simulink model "bh_zaz"  (R2016b)
settings: Solver=ode23s  StartTime=0.0  StopTime=15  RelTol=1e-5  EnableMultiTasking=on
undefined symbols (not defined in the file or in its folder): b1_damp, b2_damp, g, I1g, I2g, L1x, L1y, L1z, L2x, L2y, L2z, mass1, mass2, theta1_0, theta1_dot_0, theta2_0, theta2_dot_0, X, Y, Z
libraries: sm_lib x11, nesl_utility x10
settings Model: Creator=bhorton  LastModifiedBy=bhorton
settings SolverCC: ZeroCrossAlgorithm=Adaptive
settings OptimizationCC: LifeSpan=inf
settings DebuggingCC: SFUnexpectedBacktrackingDiag=warning  SFNoUnconditionalDefaultTransitionDiag=warning  SFExecutionAtInitializationDiag=none
settings GRTTargetCC: TargetLangStandard=C89/C90 (ANSI)
settings ConfigComp: CovMetricSettings=dw  CovHtmlReporting=on  CovSaveCumulativeToWorkspaceVar=on  CovSaveSingleToWorkspaceVar=on  CovExternalEMLEnable=off
settings SimscapeCC: SimscapeLogType=all  SimscapeLogDataHistory=10000

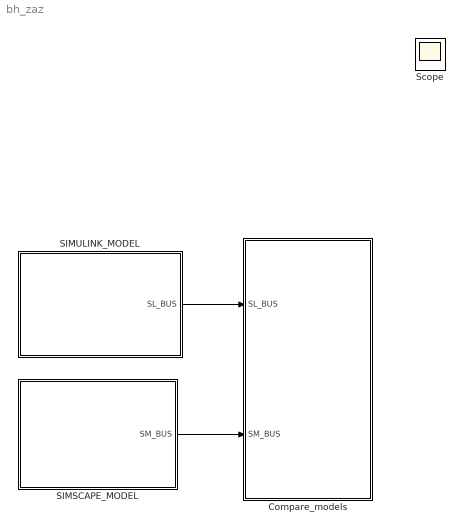
== system bh_zaz ==
  Compare_models : Subsystem
  SIMSCAPE_MODEL : Subsystem
  SIMULINK_MODEL : Subsystem
  Scope : Scope
  wires:
  SIMULINK_MODEL/1(SL_BUS) -> Compare_models/1(SL_BUS)
  SIMSCAPE_MODEL/1(SM_BUS) -> Compare_models/2(SM_BUS)

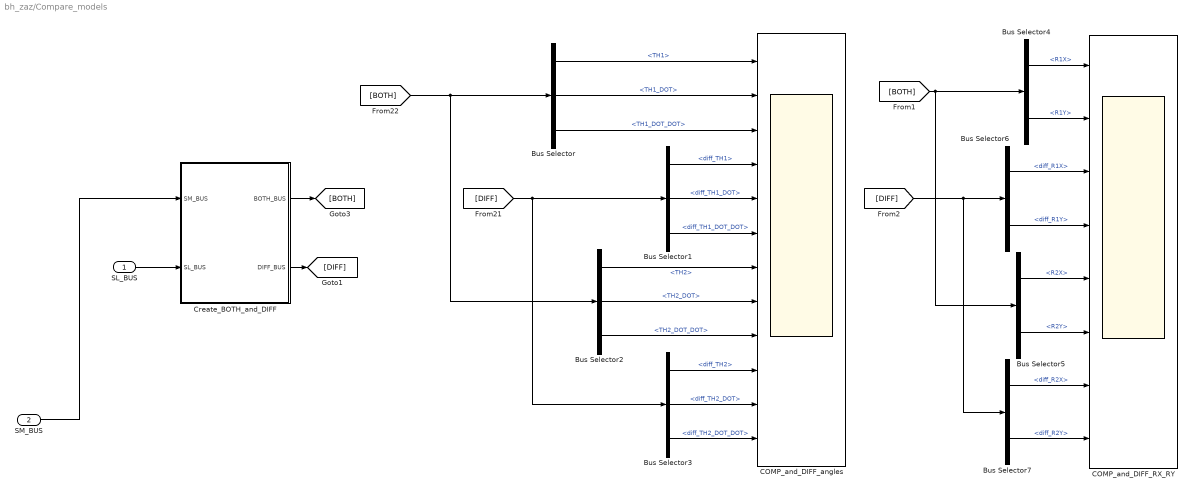
== system bh_zaz/Compare_models ==
  SL_BUS : Inport
  SM_BUS : Inport  Port=2
  Bus Selector : BusSelector  OutputSignals=TH1,TH1_DOT,TH1_DOT_DOT
  Bus Selector1 : BusSelector  OutputSignals=diff_TH1,diff_TH1_DOT,diff_TH1_DOT_DOT
  Bus Selector2 : BusSelector  OutputSignals=TH2,TH2_DOT,TH2_DOT_DOT
  Bus Selector3 : BusSelector  OutputSignals=diff_TH2,diff_TH2_DOT,diff_TH2_DOT_DOT
  Bus Selector4 : BusSelector  OutputSignals=R1X,R1Y
  Bus Selector5 : BusSelector  OutputSignals=R2X,R2Y
  Bus Selector6 : BusSelector  OutputSignals=diff_R1X,diff_R1Y
  Bus Selector7 : BusSelector  OutputSignals=diff_R2X,diff_R2Y
  COMP_and_DIFF_RX_RY : Scope  NumInputPorts=8
  COMP_and_DIFF_angles : Scope  NumInputPorts=12
  Create_BOTH_and_DIFF : Subsystem
  wires:
  SM_BUS/1 -> Create_BOTH_and_DIFF/1(SM_BUS)
  Bus Selector/3 -> COMP_and_DIFF_angles/3  "<TH1_DOT_DOT>"
  Bus Selector/2 -> COMP_and_DIFF_angles/2  "<TH1_DOT>"
  Bus Selector/1 -> COMP_and_DIFF_angles/1  "<TH1>"
  SL_BUS/1 -> Create_BOTH_and_DIFF/2(SL_BUS)
  Bus Selector1/1 -> COMP_and_DIFF_angles/4  "<diff_TH1>"
  Bus Selector1/2 -> COMP_and_DIFF_angles/5  "<diff_TH1_DOT>"
  Bus Selector1/3 -> COMP_and_DIFF_angles/6  "<diff_TH1_DOT_DOT>"
  Bus Selector2/1 -> COMP_and_DIFF_angles/7  "<TH2>"
  Bus Selector2/2 -> COMP_and_DIFF_angles/8  "<TH2_DOT>"
  Bus Selector2/3 -> COMP_and_DIFF_angles/9  "<TH2_DOT_DOT>"
  Bus Selector3/1 -> COMP_and_DIFF_angles/10  "<diff_TH2>"
  Bus Selector3/2 -> COMP_and_DIFF_angles/11  "<diff_TH2_DOT>"
  Bus Selector3/3 -> COMP_and_DIFF_angles/12  "<diff_TH2_DOT_DOT>"
  Create_BOTH_and_DIFF/1(BOTH_BUS) -> [BOTH]
  Create_BOTH_and_DIFF/2(DIFF_BUS) -> [DIFF]
  [BOTH] -> Bus Selector2/1, Bus Selector/1
  [DIFF] -> Bus Selector1/1, Bus Selector3/1
  Bus Selector4/2 -> COMP_and_DIFF_RX_RY/2  "<R1Y>"
  Bus Selector4/1 -> COMP_and_DIFF_RX_RY/1  "<R1X>"
  [BOTH] -> Bus Selector4/1, Bus Selector5/1
  Bus Selector5/1 -> COMP_and_DIFF_RX_RY/5  "<R2X>"
  Bus Selector5/2 -> COMP_and_DIFF_RX_RY/6  "<R2Y>"
  [DIFF] -> Bus Selector7/1, Bus Selector6/1
  Bus Selector6/1 -> COMP_and_DIFF_RX_RY/3  "<diff_R1X>"
  Bus Selector6/2 -> COMP_and_DIFF_RX_RY/4  "<diff_R1Y>"
  Bus Selector7/1 -> COMP_and_DIFF_RX_RY/7  "<diff_R2X>"
  Bus Selector7/2 -> COMP_and_DIFF_RX_RY/8  "<diff_R2Y>"

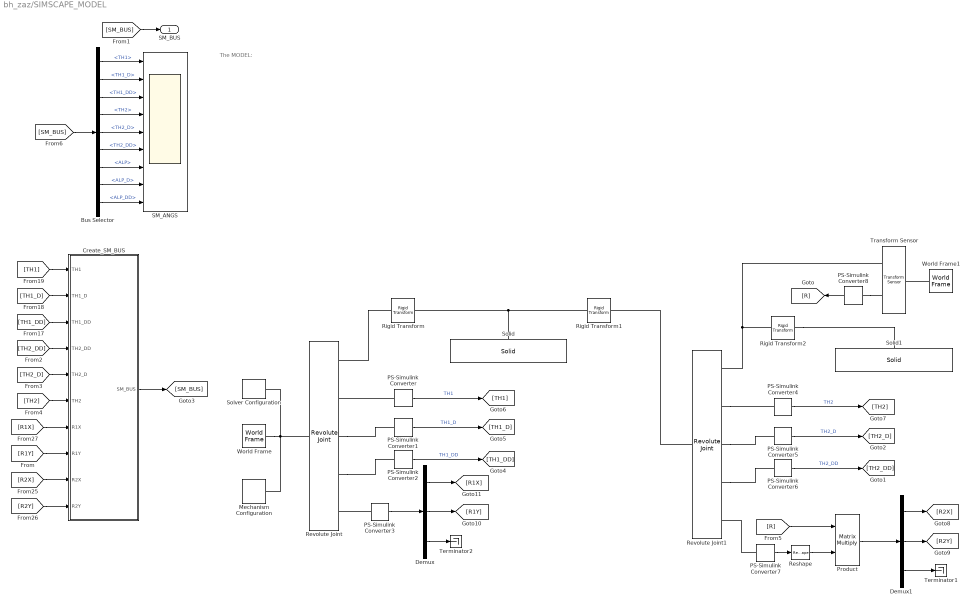
== system bh_zaz/SIMSCAPE_MODEL ==
  note: The MODEL:
  Bus Selector : BusSelector  OutputSignals=TH1,TH1_D,TH1_DD,TH2,TH2_D,TH2_DD,ALP,ALP_D,ALP_DD
  Create_SM_BUS : Subsystem
  Demux : Demux  Outputs=3
  Demux1 : Demux  Outputs=3
  Mechanism Configuration : sm_lib/Utilities/Mechanism Configuration  UniformGravity=Constant  GravityVector=[0 -9.80665 0 ]  GravityUnits=m/s^2  LinearizationDelta=0.001
  PS-Simulink Converter : nesl_utility/PS-Simulink Converter  PhysicalDomain=network_engine_domain  SubClassName=ps_output  LeftPortType=input  RightPortType=output  PseudoPeriodic=off  Frequencies=[]  Unit=rad  AffineConversion=off
  PS-Simulink Converter1 : nesl_utility/PS-Simulink Converter  PhysicalDomain=network_engine_domain  SubClassName=ps_output  LeftPortType=input  RightPortType=output  PseudoPeriodic=off  Frequencies=[]  Unit=rad/s  AffineConversion=off
  PS-Simulink Converter2 : nesl_utility/PS-Simulink Converter  PhysicalDomain=network_engine_domain  SubClassName=ps_output  LeftPortType=input  RightPortType=output  PseudoPeriodic=off  Frequencies=[]  Unit=rad/s^2  AffineConversion=off
  PS-Simulink Converter3 : nesl_utility/PS-Simulink Converter  PhysicalDomain=network_engine_domain  SubClassName=ps_output  LeftPortType=input  RightPortType=output  PseudoPeriodic=off  Frequencies=[]  Unit=N  AffineConversion=off
  PS-Simulink Converter4 : nesl_utility/PS-Simulink Converter  PhysicalDomain=network_engine_domain  SubClassName=ps_output  LeftPortType=input  RightPortType=output  PseudoPeriodic=off  Frequencies=[]  Unit=rad  AffineConversion=off
  PS-Simulink Converter5 : nesl_utility/PS-Simulink Converter  PhysicalDomain=network_engine_domain  SubClassName=ps_output  LeftPortType=input  RightPortType=output  PseudoPeriodic=off  Frequencies=[]  Unit=rad/s  AffineConversion=off
  PS-Simulink Converter6 : nesl_utility/PS-Simulink Converter  PhysicalDomain=network_engine_domain  SubClassName=ps_output  LeftPortType=input  RightPortType=output  PseudoPeriodic=off  Frequencies=[]  Unit=rad/s^2  AffineConversion=off
  PS-Simulink Converter7 : nesl_utility/PS-Simulink Converter  PhysicalDomain=network_engine_domain  SubClassName=ps_output  LeftPortType=input  RightPortType=output  PseudoPeriodic=off  Frequencies=[]  Unit=N  AffineConversion=off
  PS-Simulink Converter8 : nesl_utility/PS-Simulink Converter  PhysicalDomain=network_engine_domain  SubClassName=ps_output  LeftPortType=input  RightPortType=output  PseudoPeriodic=off  Frequencies=[]  Unit=1  AffineConversion=off
  Product : Product  Multiplication=Matrix(*)
  Reshape : Reshape  OutputDimensionality=Column vector (2-D)
  Revolute Joint : sm_lib/Joints/Revolute Joint  SenseConstraintForce=on  SenseConstraintForceX=off  SenseConstraintForceY=off  SenseConstraintForceZ=off  SenseConstraintTorque=off  SenseConstraintTorqueX=off  SenseConstraintTorqueY=off  SenseConstraintTorqueZ=off  SenseTotalForce=off  SenseTotalForceX=off  SenseTotalForceY=off  SenseTotalForceZ=off  SenseTotalTorque=off  SenseTotalTorqueX=off  SenseTotalTorqueY=off  SenseTotalTorqueZ=off  CompositeWrenchDir=BaseOnFollower  CompositeWrenchFrame=BaseFrame  EquilibriumPosition=0  EquilibriumPositionUnits=deg  SpringStiffness=0  SpringStiffnessUnits=N*m/deg  DampingCoefficient=b1_damp  DampingCoefficientUnits=N*m/(rad/s)  TorqueActuationMode=NoTorque  MotionActuationMode=ComputedMotion  SensePosition=on  SenseVelocity=on  SenseAcceleration=on  SenseTorqueForce=off  PositionTargetSpecify=on  PositionTargetPriority=Low  PositionTargetValue=theta1_0  PositionTargetValueUnits=rad  VelocityTargetSpecify=on  VelocityTargetPriority=High  VelocityTargetValue=theta1_dot_0  VelocityTargetValueUnits=rad/s
  Revolute Joint1 : sm_lib/Joints/Revolute Joint  SenseConstraintForce=on  SenseConstraintForceX=off  SenseConstraintForceY=off  SenseConstraintForceZ=off  SenseConstraintTorque=off  SenseConstraintTorqueX=off  SenseConstraintTorqueY=off  SenseConstraintTorqueZ=off  SenseTotalForce=off  SenseTotalForceX=off  SenseTotalForceY=off  SenseTotalForceZ=off  SenseTotalTorque=off  SenseTotalTorqueX=off  SenseTotalTorqueY=off  SenseTotalTorqueZ=off  CompositeWrenchDir=BaseOnFollower  CompositeWrenchFrame=FollowerFrame  EquilibriumPosition=0  EquilibriumPositionUnits=deg  SpringStiffness=0  SpringStiffnessUnits=N*m/deg  DampingCoefficient=b2_damp  DampingCoefficientUnits=N*m/(rad/s)  TorqueActuationMode=NoTorque  MotionActuationMode=ComputedMotion  SensePosition=on  SenseVelocity=on  SenseAcceleration=on  SenseTorqueForce=off  PositionTargetSpecify=on  PositionTargetPriority=Low  PositionTargetValue=theta2_0  PositionTargetValueUnits=rad  VelocityTargetSpecify=on  VelocityTargetPriority=High  VelocityTargetValue=theta2_dot_0  VelocityTargetValueUnits=rad/s
  Rigid Transform : sm_lib/Frames and Transforms/Rigid Transform  TranslationMethod=StandardAxis  TranslationStandardOffset=L1x/2  TranslationLengthUnit=m  TranslationStandardAxis=+X  TranslationCartesianOffset=[0 0 0]  TranslationROffset=0  TranslationROffsetUnits=m  TranslationZOffset=0  TranslationZOffsetUnits=m  TranslationThetaOffset=0  TranslationThetaOffsetUnits=deg  RotationMethod=None  RotationAngleUnits=deg  RotationStandardAxis=+Z  RotationAngle=0.0  RotationArbitraryAxis=[0 0 1]  FollAlignAxisA=+X  BaseAlignAxisA=+Y  FollAlignAxisB=+Y  BaseAlignAxisB=+Z  RotationSequenceAxes=FollowerAxes  RotationSequence=XYX  RotationSequenceAngles=[0 0 0]  RotationSequenceAnglesUnits=deg  RotationMatrix=[1 0 0; 0 1 0; 0 0 1]
  Rigid Transform1 : sm_lib/Frames and Transforms/Rigid Transform  TranslationMethod=StandardAxis  TranslationStandardOffset=L1x/2  TranslationLengthUnit=m  TranslationStandardAxis=+X  TranslationCartesianOffset=[0 0 0]  TranslationROffset=0  TranslationROffsetUnits=m  TranslationZOffset=0  TranslationZOffsetUnits=m  TranslationThetaOffset=0  TranslationThetaOffsetUnits=deg  RotationMethod=None  RotationAngleUnits=deg  RotationStandardAxis=+Z  RotationAngle=0.0  RotationArbitraryAxis=[0 0 1]  FollAlignAxisA=+X  BaseAlignAxisA=+Y  FollAlignAxisB=+Y  BaseAlignAxisB=+Z  RotationSequenceAxes=FollowerAxes  RotationSequence=XYX  RotationSequenceAngles=[0 0 0]  RotationSequenceAnglesUnits=deg  RotationMatrix=[1 0 0; 0 1 0; 0 0 1]
  Rigid Transform2 : sm_lib/Frames and Transforms/Rigid Transform  TranslationMethod=StandardAxis  TranslationStandardOffset=L2x/2  TranslationLengthUnit=m  TranslationStandardAxis=+X  TranslationCartesianOffset=[0 0 0]  TranslationROffset=0  TranslationROffsetUnits=m  TranslationZOffset=0  TranslationZOffsetUnits=m  TranslationThetaOffset=0  TranslationThetaOffsetUnits=deg  RotationMethod=None  RotationAngleUnits=deg  RotationStandardAxis=+Z  RotationAngle=0.0  RotationArbitraryAxis=[0 0 1]  FollAlignAxisA=+X  BaseAlignAxisA=+Y  FollAlignAxisB=+Y  BaseAlignAxisB=+Z  RotationSequenceAxes=FollowerAxes  RotationSequence=XYX  RotationSequenceAngles=[0 0 0]  RotationSequenceAnglesUnits=deg  RotationMatrix=[1 0 0; 0 1 0; 0 0 1]
  SM_ANGS : Scope  NumInputPorts=9
  Solid : sm_lib/Body Elements/Solid  InertiaType=CalculateFromGeometry  Mass=1  MassUnits=kg  CenterOfMass=[0 0 0]  CenterOfMassUnits=m  MomentsOfInertia=[1 1 1]  MomentsOfInertiaUnits=kg*m^2  ProductsOfInertia=[0 0 0]  ProductsOfInertiaUnits=kg*m^2  DensityBased=on  Density=density  DensityUnits=kg/(m^3)  DoExposeReferenceFrame=on  SerializedFrames=<Frames/>  GraphicType=FromGeometry  MarkerShape=Sphere  MarkerSize=10  GraphicVisPropType=SimpleVisualProperties  GraphicDiffuseColor=[0.8 0.8 1.0]  GraphicSpecularColor=[0.5 0.5 0.5 1.0]  GraphicAmbientColor=[0.15 0.15 0.15 1.0]  GraphicEmissiveColor=[0.0 0.0 0.0 1.0]  GraphicShininess=75  GraphicOpacity=1.0  GeometryShape=Brick  RectangleSize=[1 1]  RectangleSizeUnits=m  BrickDimensions=[L1x, L1y, L1z ]  BrickDimensionUnits=m  CylinderRadius=1  CylinderRadiusUnits=m  CylinderLength=1  CylinderLengthUnits=m  SphereRadius=1  SphereRadiusUnits=m  EllipsoidRadii=[1 1 1]  EllipsoidRadiiUnits=m  ExtrusionCrossSection=[1 1; -1 1; -1 -1; 1 -1]  ExtrusionCrossSectionUnits=m  ExtrusionLength=1  ExtrusionLengthUnits=m  PolygonNumSides=3  PolygonOuterRadius=1  PolygonOuterRadiusUnits=m  ExtGeomFileType=STEP  ExtGeomFileUnits=m  RevolutionCrossSection=[1 1; 1 -1; 2 -1; 2 1]  RevolutionCrossSectionUnits=m  RevolutionExtent=Full  RevolutionAngle=180  RevolutionAngleUnits=deg
  Solid1 : sm_lib/Body Elements/Solid  InertiaType=CalculateFromGeometry  Mass=1  MassUnits=kg  CenterOfMass=[0 0 0]  CenterOfMassUnits=m  MomentsOfInertia=[1 1 1]  MomentsOfInertiaUnits=kg*m^2  ProductsOfInertia=[0 0 0]  ProductsOfInertiaUnits=kg*m^2  DensityBased=on  Density=density  DensityUnits=kg/(m^3)  DoExposeReferenceFrame=on  SerializedFrames=<Frames/>  GraphicType=FromGeometry  MarkerShape=Sphere  MarkerSize=10  GraphicVisPropType=SimpleVisualProperties  GraphicDiffuseColor=[1.0 0.6 1.0]  GraphicSpecularColor=[0.5 0.5 0.5 1.0]  GraphicAmbientColor=[0.15 0.15 0.15 1.0]  GraphicEmissiveColor=[0.0 0.0 0.0 1.0]  GraphicShininess=75  GraphicOpacity=1.0  GeometryShape=Brick  RectangleSize=[1 1]  RectangleSizeUnits=m  BrickDimensions=[L2x, L2y, L2z ]  BrickDimensionUnits=m  CylinderRadius=1  CylinderRadiusUnits=m  CylinderLength=1  CylinderLengthUnits=m  SphereRadius=1  SphereRadiusUnits=m  EllipsoidRadii=[1 1 1]  EllipsoidRadiiUnits=m  ExtrusionCrossSection=[1 1; -1 1; -1 -1; 1 -1]  ExtrusionCrossSectionUnits=m  ExtrusionLength=1  ExtrusionLengthUnits=m  PolygonNumSides=3  PolygonOuterRadius=1  PolygonOuterRadiusUnits=m  ExtGeomFileType=STEP  ExtGeomFileUnits=m  RevolutionCrossSection=[1 1; 1 -1; 2 -1; 2 1]  RevolutionCrossSectionUnits=m  RevolutionExtent=Full  RevolutionAngle=180  RevolutionAngleUnits=deg
  Solver Configuration : nesl_utility/Solver Configuration  PhysicalDomain=network_engine_domain  SubClassName=solver  LeftPortType=input  RightPortType=generic  Accelerate=off  Tones=[]  Harmonics=[]  SimulateNoise=off  Profile=off  UseLocalSampling=off  EnableSwitchedLinearOptims=on  FrequencyDomain=off  UseCCode=off  RelTol=0.001  AbsTol=1e-06  MinStep=1e-09  ToWorkspace=off  RevertToSquareIcSolve=off  NumHomotopyIterations=100  PhasorMode=off  PhasorModeNumHarmonics=1  OverrideAbsTol=off  DoDC=off  ResidualTolerance=1e-09  UseLocalSolver=off  LocalSolverChoice=NE_BACKWARD_EULER_ADVANCER  LocalSolverSampleTime=0.001  DoFixedCost=off  MaxNonlinIter=3  MaxModeIter=2  LinearAlgebra=Sparse  DelaysMemoryBudget=1024  AutomaticFiltering=on  FilteringTimeConstant=0.001
  Terminator1 : Terminator
  Terminator2 : Terminator
  Transform Sensor : sm_lib/Frames and Transforms/Transform Sensor  MeasurementFrame=World  SenseAngle=off  SenseAxis=off  SenseAngle1=off  SenseAngle2=off  SenseAngle3=off  SenseQ=off  SenseR=on  SenseOmegaX=off  SenseOmegaY=off  SenseOmegaZ=off  SenseOmega1=off  SenseOmega2=off  SenseOmega3=off  SenseQDot=off  SenseRDot=off  SenseAlphaX=off  SenseAlphaY=off  SenseAlphaZ=off  SenseAlpha1=off  SenseAlpha2=off  SenseAlpha3=off  SenseQDDot=off  SenseRDDot=off  SenseX=off  SenseY=off  SenseZ=off  SenseRad=off  SenseAzim=off  SenseDist=off  SenseInc=off  SenseXDot=off  SenseYDot=off  SenseZDot=off  SenseRadDot=off  SenseAzimDot=off  SenseDistDot=off  SenseIncDot=off  SenseXDDot=off  SenseYDDot=off  SenseZDDot=off  SenseRadDDot=off  SenseAzimDDot=off  SenseDistDDot=off  SenseIncDDot=off
  World Frame : sm_lib/Frames and Transforms/World Frame
  World Frame1 : sm_lib/Frames and Transforms/World Frame
  SM_BUS : Outport
  wires:
  PS-Simulink Converter/1 -> [TH1]  "TH1"
  PS-Simulink Converter2/1 -> [TH1_DD]  "TH1_DD"
  PS-Simulink Converter1/1 -> [TH1_D]  "TH1_D"
  PS-Simulink Converter3/1 -> Demux/1
  [SM_BUS] -> SM_BUS/1
  PS-Simulink Converter4/1 -> [TH2]  "TH2"
  PS-Simulink Converter6/1 -> [TH2_DD]  "TH2_DD"
  PS-Simulink Converter5/1 -> [TH2_D]  "TH2_D"
  PS-Simulink Converter7/1 -> Reshape/1
  [TH2_D] -> Create_SM_BUS/5(TH2_D)
  [TH1_D] -> Create_SM_BUS/2(TH1_D)
  [TH2_DD] -> Create_SM_BUS/4(TH2_DD)
  [TH2] -> Create_SM_BUS/6(TH2)
  [TH1_DD] -> Create_SM_BUS/3(TH1_DD)
  [TH1] -> Create_SM_BUS/1(TH1)
  Create_SM_BUS/1(SM_BUS) -> [SM_BUS]
  [SM_BUS] -> Bus Selector/1
  Bus Selector/2 -> SM_ANGS/2  "<TH1_D>"
  Bus Selector/3 -> SM_ANGS/3  "<TH1_DD>"
  Bus Selector/1 -> SM_ANGS/1  "<TH1>"
  Bus Selector/4 -> SM_ANGS/4  "<TH2>"
  Bus Selector/5 -> SM_ANGS/5  "<TH2_D>"
  Bus Selector/6 -> SM_ANGS/6  "<TH2_DD>"
  Bus Selector/7 -> SM_ANGS/7  "<ALP>"
  Bus Selector/8 -> SM_ANGS/8  "<ALP_D>"
  Bus Selector/9 -> SM_ANGS/9  "<ALP_DD>"
  Demux/2 -> [R1Y]
  Demux/1 -> [R1X]
  [R1X] -> Create_SM_BUS/7(R1X)
  [R1Y] -> Create_SM_BUS/8(R1Y)
  [R2X] -> Create_SM_BUS/9(R2X)
  [R2Y] -> Create_SM_BUS/10(R2Y)
  Demux/3 -> Terminator2/1
  Demux1/1 -> [R2X]
  Demux1/2 -> [R2Y]
  Demux1/3 -> Terminator1/1
  PS-Simulink Converter8/1 -> [R]
  Reshape/1 -> Product/2
  [R] -> Product/1
  Product/1 -> Demux1/1
  connections:
  World Frame/RConn1 -- Revolute Joint/LConn1 -- Solver Configuration/RConn1 -- Mechanism Configuration/RConn1
  PS-Simulink Converter3/LConn1 -- Revolute Joint/RConn5
  Solid/RConn1 -- Rigid Transform1/LConn1 -- Rigid Transform/RConn1
  Revolute Joint/RConn3 -- PS-Simulink Converter1/LConn1
  Revolute Joint/RConn4 -- PS-Simulink Converter2/LConn1
  Rigid Transform/LConn1 -- Revolute Joint/RConn1
  PS-Simulink Converter/LConn1 -- Revolute Joint/RConn2
  Revolute Joint1/LConn1 -- Rigid Transform1/RConn1
  Revolute Joint1/RConn3 -- PS-Simulink Converter5/LConn1
  Revolute Joint1/RConn2 -- PS-Simulink Converter4/LConn1
  Revolute Joint1/RConn4 -- PS-Simulink Converter6/LConn1
  PS-Simulink Converter7/LConn1 -- Revolute Joint1/RConn5
  Rigid Transform2/RConn1 -- Solid1/RConn1
  Rigid Transform2/LConn1 -- Transform Sensor/RConn1 -- Revolute Joint1/RConn1
  World Frame1/RConn1 -- Transform Sensor/LConn1
  PS-Simulink Converter8/LConn1 -- Transform Sensor/RConn2

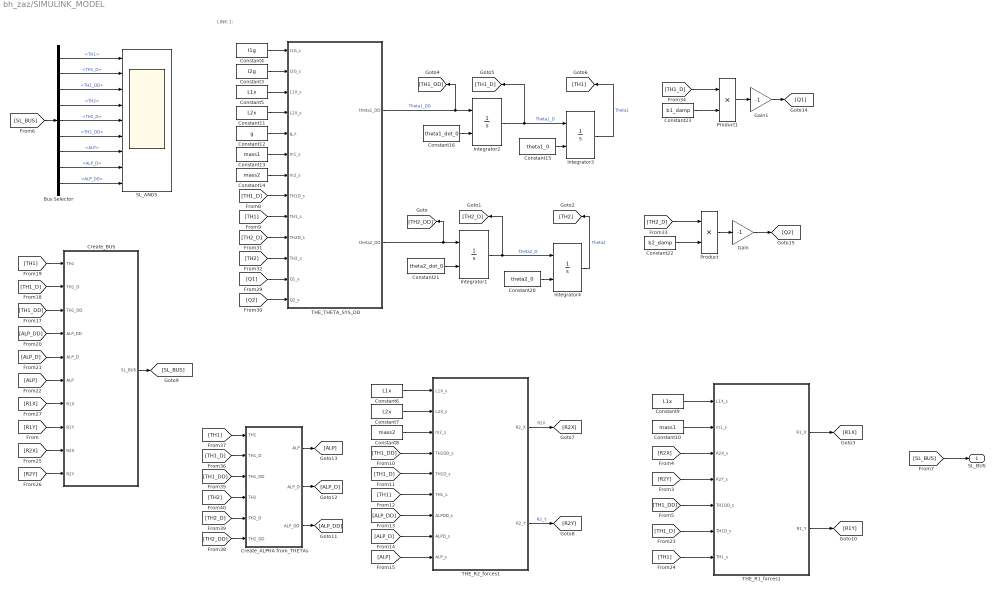
== system bh_zaz/SIMULINK_MODEL ==
  note: LINK 1:
  Bus Selector : BusSelector  OutputSignals=TH1,TH1_D,TH1_DD,TH2,TH2_D,TH2_DD,ALP,ALP_D,ALP_DD
  Constant10 : Constant  Value=mass1
  Constant11 : Constant  Value=L2x
  Constant12 : Constant  Value=g
  Constant13 : Constant  Value=mass1
  Constant14 : Constant  Value=mass2
  Constant15 : Constant  Value=theta1_0
  Constant16 : Constant  Value=theta1_dot_0
  Constant20 : Constant  Value=theta2_0
  Constant21 : Constant  Value=theta2_dot_0
  Constant22 : Constant  Value=b2_damp
  Constant23 : Constant  Value=b1_damp
  Constant3 : Constant  Value=I2g
  Constant4 : Constant  Value=I1g
  Constant5 : Constant  Value=L1x
  Constant6 : Constant  Value=L1x
  Constant7 : Constant  Value=L2x
  Constant8 : Constant  Value=mass2
  Constant9 : Constant  Value=L1x
  Create_ALPHA from_THETAs : Subsystem
  Create_BUS : Subsystem
  Gain : Gain  Gain=-1
  Gain1 : Gain  Gain=-1
  Integrator{1..4} (4 alike) : Integrator  InitialConditionSource=external
  Product : Product
  Product1 : Product
  SL_ANGS : Scope  NumInputPorts=9
  THE_R1_forces1 : MATLAB Function  TreatAsAtomicUnit=on
  THE_R2_forces1 : MATLAB Function  TreatAsAtomicUnit=on
  THE_THETA_SYS_DD : MATLAB Function  TreatAsAtomicUnit=on
  SL_BUS : Outport
  wires:
  [SL_BUS] -> Bus Selector/1
  [SL_BUS] -> SL_BUS/1
  Constant6/1 -> THE_R2_forces1/1(L1X_s)
  Constant7/1 -> THE_R2_forces1/2(L2X_s)
  Constant8/1 -> THE_R2_forces1/3(m2_s)
  [ALP_DD] -> THE_R2_forces1/7(ALPDD_s)
  [ALP_D] -> THE_R2_forces1/8(ALPD_s)
  [ALP] -> THE_R2_forces1/9(ALP_s)
  [TH1] -> THE_R2_forces1/6(TH1_s)
  [TH1_D] -> THE_R2_forces1/5(TH1D_s)
  [TH1_DD] -> THE_R2_forces1/4(TH1DD_s)
  THE_R2_forces1/2(R2_Y) -> [R2Y]  "R2_Y"
  THE_R2_forces1/1(R2_X) -> [R2X]  "R2X"
  [ALP_D] -> Create_BUS/5(ALP_D)
  [TH1_D] -> Create_BUS/2(TH1_D)
  [ALP_DD] -> Create_BUS/4(ALP_DD)
  [ALP] -> Create_BUS/6(ALP)
  [TH1_DD] -> Create_BUS/3(TH1_DD)
  [TH1] -> Create_BUS/1(TH1)
  Create_BUS/1(SL_BUS) -> [SL_BUS]
  Bus Selector/2 -> SL_ANGS/2  "<TH1_D>"
  Bus Selector/3 -> SL_ANGS/3  "<TH1_DD>"
  Bus Selector/1 -> SL_ANGS/1  "<TH1>"
  Bus Selector/4 -> SL_ANGS/4  "<TH2>"
  Bus Selector/5 -> SL_ANGS/5  "<TH2_D>"
  Bus Selector/6 -> SL_ANGS/6  "<TH2_DD>"
  Bus Selector/7 -> SL_ANGS/7  "<ALP>"
  Bus Selector/8 -> SL_ANGS/8  "<ALP_D>"
  Bus Selector/9 -> SL_ANGS/9  "<ALP_DD>"
  Constant9/1 -> THE_R1_forces1/1(L1X_s)
  Constant10/1 -> THE_R1_forces1/2(m1_s)
  [R2X] -> THE_R1_forces1/3(R2X_s)
  [R2Y] -> THE_R1_forces1/4(R2Y_s)
  [TH1] -> THE_R1_forces1/7(TH1_s)
  [TH1_D] -> THE_R1_forces1/6(TH1D_s)
  [TH1_DD] -> THE_R1_forces1/5(TH1DD_s)
  THE_R1_forces1/2(R1_Y) -> [R1Y]
  THE_R1_forces1/1(R1_X) -> [R1X]
  [R1X] -> Create_BUS/7(R1X)
  [R1Y] -> Create_BUS/8(R1Y)
  [R2Y] -> Create_BUS/10(R2Y)
  [R2X] -> Create_BUS/9(R2X)
  Constant4/1 -> THE_THETA_SYS_DD/1(I1G_s)
  Constant3/1 -> THE_THETA_SYS_DD/2(I2G_s)
  Constant11/1 -> THE_THETA_SYS_DD/4(L2X_s)
  Constant5/1 -> THE_THETA_SYS_DD/3(L1X_s)
  Constant12/1 -> THE_THETA_SYS_DD/5(g_s)
  Constant13/1 -> THE_THETA_SYS_DD/6(m1_s)
  Constant14/1 -> THE_THETA_SYS_DD/7(m2_s)
  [TH1] -> THE_THETA_SYS_DD/9(TH1_s)
  THE_THETA_SYS_DD/1(theta1_DD) -> [TH1_DD], Integrator2/1  "Theta1_DD"
  Integrator2/1 -> [TH1_D], Integrator3/1  "Theta1_D"
  Constant15/1 -> Integrator3/2
  Constant16/1 -> Integrator2/2
  Integrator3/1 -> [TH1]  "Theta1"
  Integrator1/1 -> [TH2_D], Integrator4/1  "Theta2_D"
  Constant20/1 -> Integrator4/2
  Constant21/1 -> Integrator1/2
  Integrator4/1 -> [TH2]  "Theta2"
  [TH2] -> THE_THETA_SYS_DD/11(TH2_s)
  [TH2_D] -> THE_THETA_SYS_DD/10(TH2D_s)
  Product/1 -> Gain/1
  [TH2_D] -> Product/1
  Constant22/1 -> Product/2
  Product1/1 -> Gain1/1
  [TH1_D] -> Product1/1
  Constant23/1 -> Product1/2
  [TH1_D] -> Create_ALPHA from_THETAs/2(TH1_D)
  [TH1_DD] -> Create_ALPHA from_THETAs/3(TH1_DD)
  [TH1] -> Create_ALPHA from_THETAs/1(TH1)
  [TH2] -> Create_ALPHA from_THETAs/4(TH2)
  [TH2_D] -> Create_ALPHA from_THETAs/5(TH2_D)
  [TH2_DD] -> Create_ALPHA from_THETAs/6(TH2_DD)
  Create_ALPHA from_THETAs/2(ALP_D) -> [ALP_D]
  Create_ALPHA from_THETAs/3(ALP_DD) -> [ALP_DD]
  Create_ALPHA from_THETAs/1(ALP) -> [ALP]
  [TH1_D] -> THE_THETA_SYS_DD/8(TH1D_s)
  THE_THETA_SYS_DD/2(theta2_DD) -> [TH2_DD], Integrator1/1
  [Q1] -> THE_THETA_SYS_DD/12(Q1_s)
  [Q2] -> THE_THETA_SYS_DD/13(Q2_s)
  Gain1/1 -> [Q1]
  Gain/1 -> [Q2]

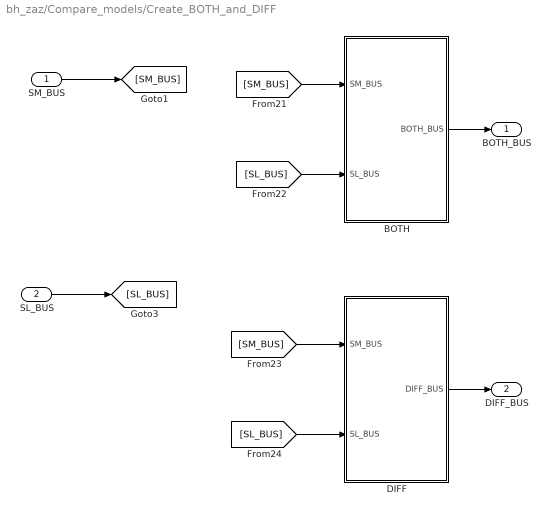
== system bh_zaz/Compare_models/Create_BOTH_and_DIFF ==
  SM_BUS : Inport
  SL_BUS : Inport  Port=2
  BOTH : Subsystem
  DIFF : Subsystem
  BOTH_BUS : Outport
  DIFF_BUS : Outport  Port=2
  wires:
  SL_BUS/1 -> [SL_BUS]
  SM_BUS/1 -> [SM_BUS]
  [SM_BUS] -> BOTH/1(SM_BUS)
  [SL_BUS] -> BOTH/2(SL_BUS)
  [SM_BUS] -> DIFF/1(SM_BUS)
  [SL_BUS] -> DIFF/2(SL_BUS)
  DIFF/1(DIFF_BUS) -> DIFF_BUS/1
  BOTH/1(BOTH_BUS) -> BOTH_BUS/1

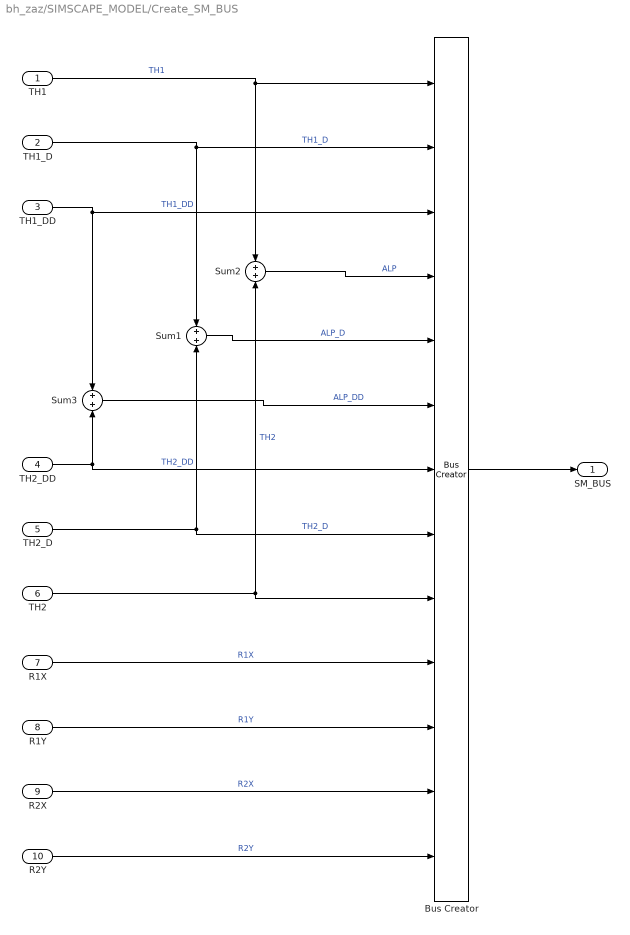
== system bh_zaz/SIMSCAPE_MODEL/Create_SM_BUS ==
  TH1 : Inport
  TH1_D : Inport  Port=2
  TH1_DD : Inport  Port=3
  TH2_DD : Inport  Port=4
  TH2_D : Inport  Port=5
  TH2 : Inport  Port=6
  R1X : Inport  Port=7
  R1Y : Inport  Port=8
  R2X : Inport  Port=9
  R2Y : Inport  Port=10
  Bus Creator : BusCreator  Inputs=13
  Sum1 : Sum  Inputs=+|+
  Sum2 : Sum  Inputs=+|+
  Sum3 : Sum  Inputs=+|+
  SM_BUS : Outport
  wires:
  TH2_DD/1 -> Bus Creator/7, Sum3/2  "TH2_DD"
  TH1_DD/1 -> Sum3/1, Bus Creator/3  "TH1_DD"
  TH1_D/1 -> Bus Creator/2, Sum1/1  "TH1_D"
  TH2_D/1 -> Bus Creator/8, Sum1/2  "TH2_D"
  TH1/1 -> Bus Creator/1, Sum2/1  "TH1"
  TH2/1 -> Bus Creator/9, Sum2/2  "TH2"
  Sum2/1 -> Bus Creator/4  "ALP"
  Sum1/1 -> Bus Creator/5  "ALP_D"
  Sum3/1 -> Bus Creator/6  "ALP_DD"
  Bus Creator/1 -> SM_BUS/1
  R1Y/1 -> Bus Creator/11  "R1Y"
  R1X/1 -> Bus Creator/10  "R1X"
  R2Y/1 -> Bus Creator/13  "R2Y"
  R2X/1 -> Bus Creator/12  "R2X"

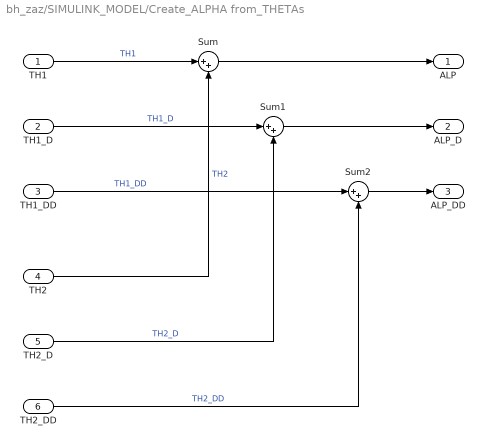
== system bh_zaz/SIMULINK_MODEL/Create_ALPHA from_THETAs ==
  TH1 : Inport
  TH1_D : Inport  Port=2
  TH1_DD : Inport  Port=3
  TH2 : Inport  Port=4
  TH2_D : Inport  Port=5
  TH2_DD : Inport  Port=6
  Sum : Sum  Inputs=|++
  Sum1 : Sum  Inputs=|++
  Sum2 : Sum  Inputs=|++
  ALP : Outport
  ALP_D : Outport  Port=2
  ALP_DD : Outport  Port=3
  wires:
  TH1_DD/1 -> Sum2/1  "TH1_DD"
  TH1_D/1 -> Sum1/1  "TH1_D"
  TH1/1 -> Sum/1  "TH1"
  TH2_DD/1 -> Sum2/2  "TH2_DD"
  TH2_D/1 -> Sum1/2  "TH2_D"
  TH2/1 -> Sum/2  "TH2"
  Sum/1 -> ALP/1
  Sum1/1 -> ALP_D/1
  Sum2/1 -> ALP_DD/1

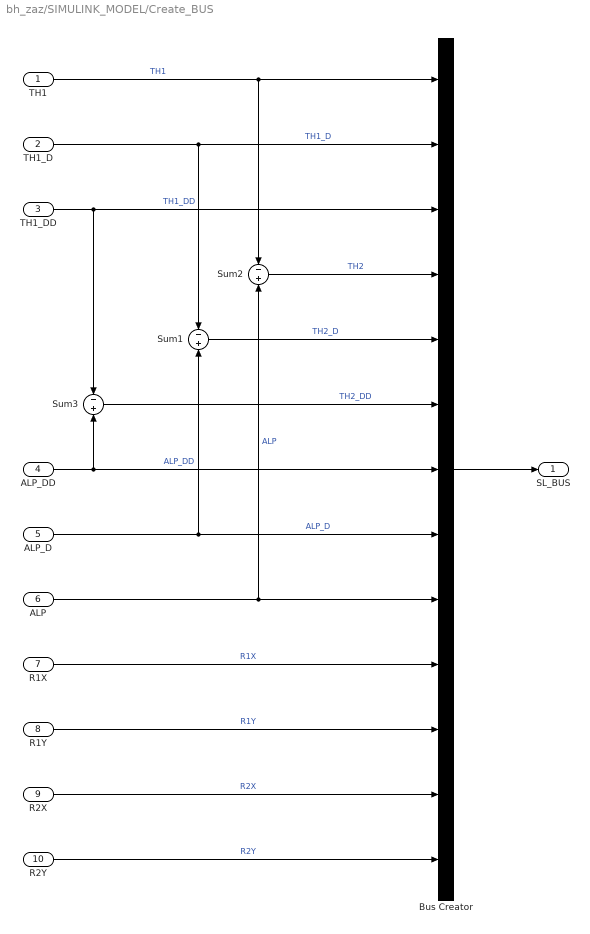
== system bh_zaz/SIMULINK_MODEL/Create_BUS ==
  TH1 : Inport
  TH1_D : Inport  Port=2
  TH1_DD : Inport  Port=3
  ALP_DD : Inport  Port=4
  ALP_D : Inport  Port=5
  ALP : Inport  Port=6
  R1X : Inport  Port=7
  R1Y : Inport  Port=8
  R2X : Inport  Port=9
  R2Y : Inport  Port=10
  Bus Creator : BusCreator  Inputs=13
  Sum1 : Sum  Inputs=-|+
  Sum2 : Sum  Inputs=-|+
  Sum3 : Sum  Inputs=-|+
  SL_BUS : Outport
  wires:
  ALP_DD/1 -> Bus Creator/7, Sum3/2  "ALP_DD"
  TH1_DD/1 -> Sum3/1, Bus Creator/3  "TH1_DD"
  TH1_D/1 -> Bus Creator/2, Sum1/1  "TH1_D"
  ALP_D/1 -> Bus Creator/8, Sum1/2  "ALP_D"
  TH1/1 -> Bus Creator/1, Sum2/1  "TH1"
  ALP/1 -> Bus Creator/9, Sum2/2  "ALP"
  Sum2/1 -> Bus Creator/4  "TH2"
  Sum1/1 -> Bus Creator/5  "TH2_D"
  Sum3/1 -> Bus Creator/6  "TH2_DD"
  Bus Creator/1 -> SL_BUS/1
  R1Y/1 -> Bus Creator/11  "R1Y"
  R1X/1 -> Bus Creator/10  "R1X"
  R2Y/1 -> Bus Creator/13  "R2Y"
  R2X/1 -> Bus Creator/12  "R2X"

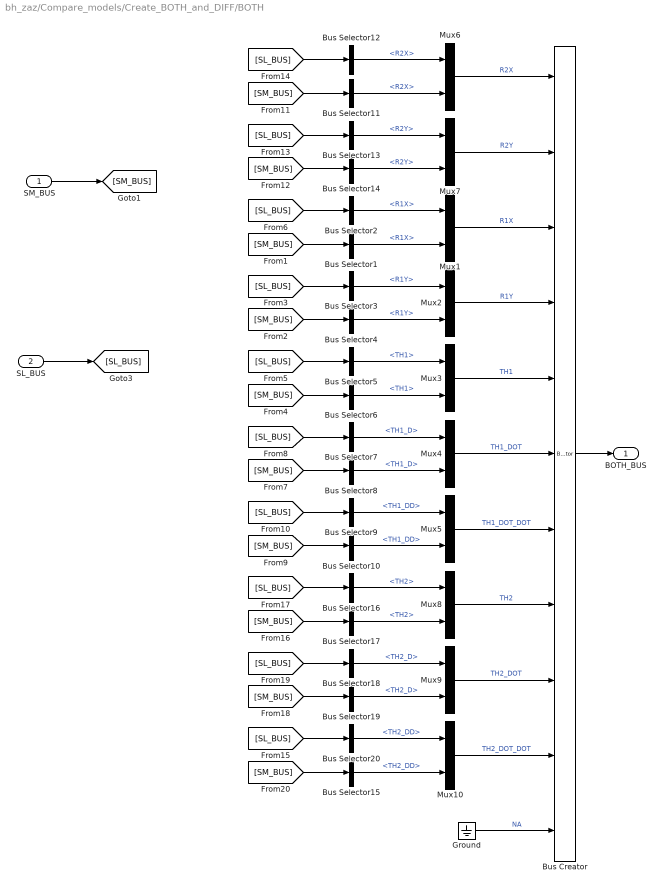
== system bh_zaz/Compare_models/Create_BOTH_and_DIFF/BOTH ==
  SM_BUS : Inport
  SL_BUS : Inport  Port=2
  Bus Creator : BusCreator  Inputs=11
  Bus Selector1 : BusSelector  OutputSignals=R1X
  Bus Selector10 : BusSelector  OutputSignals=TH1_DD
  Bus Selector11 : BusSelector  OutputSignals=R2X
  Bus Selector12 : BusSelector  OutputSignals=R2X
  Bus Selector13 : BusSelector  OutputSignals=R2Y
  Bus Selector14 : BusSelector  OutputSignals=R2Y
  Bus Selector15 : BusSelector  OutputSignals=TH2_DD
  Bus Selector16 : BusSelector  OutputSignals=TH2
  Bus Selector17 : BusSelector  OutputSignals=TH2
  Bus Selector18 : BusSelector  OutputSignals=TH2_D
  Bus Selector19 : BusSelector  OutputSignals=TH2_D
  Bus Selector2 : BusSelector  OutputSignals=R1X
  Bus Selector20 : BusSelector  OutputSignals=TH2_DD
  Bus Selector3 : BusSelector  OutputSignals=R1Y
  Bus Selector4 : BusSelector  OutputSignals=R1Y
  Bus Selector5 : BusSelector  OutputSignals=TH1
  Bus Selector6 : BusSelector  OutputSignals=TH1
  Bus Selector7 : BusSelector  OutputSignals=TH1_D
  Bus Selector8 : BusSelector  OutputSignals=TH1_D
  Bus Selector9 : BusSelector  OutputSignals=TH1_DD
  Ground : Ground
  Mux{1..10} (10 alike) : Mux  Inputs=2
  BOTH_BUS : Outport
  wires:
  SL_BUS/1 -> [SL_BUS]
  SM_BUS/1 -> [SM_BUS]
  [SL_BUS] -> Bus Selector2/1
  [SM_BUS] -> Bus Selector1/1
  [SL_BUS] -> Bus Selector3/1
  [SM_BUS] -> Bus Selector4/1
  [SM_BUS] -> Bus Selector6/1
  [SL_BUS] -> Bus Selector5/1
  [SL_BUS] -> Bus Selector7/1
  [SM_BUS] -> Bus Selector8/1
  [SL_BUS] -> Bus Selector9/1
  [SM_BUS] -> Bus Selector10/1
  Bus Selector1/1 -> Mux1/2  "<R1X>"
  Bus Selector2/1 -> Mux1/1  "<R1X>"
  Bus Selector3/1 -> Mux2/1  "<R1Y>"
  Bus Selector4/1 -> Mux2/2  "<R1Y>"
  Bus Selector5/1 -> Mux3/1  "<TH1>"
  Bus Selector6/1 -> Mux3/2  "<TH1>"
  Bus Selector7/1 -> Mux4/1  "<TH1_D>"
  Bus Selector8/1 -> Mux4/2  "<TH1_D>"
  Bus Selector9/1 -> Mux5/1  "<TH1_DD>"
  Bus Selector10/1 -> Mux5/2  "<TH1_DD>"
  Mux1/1 -> Bus Creator/3  "R1X"
  Mux2/1 -> Bus Creator/4  "R1Y"
  Mux3/1 -> Bus Creator/5  "TH1"
  Mux4/1 -> Bus Creator/6  "TH1_DOT"
  Bus Creator/1 -> BOTH_BUS/1
  Mux5/1 -> Bus Creator/7  "TH1_DOT_DOT"
  [SL_BUS] -> Bus Selector12/1
  [SM_BUS] -> Bus Selector11/1
  [SL_BUS] -> Bus Selector13/1
  Bus Selector11/1 -> Mux6/2  "<R2X>"
  Bus Selector12/1 -> Mux6/1  "<R2X>"
  Bus Selector13/1 -> Mux7/1  "<R2Y>"
  Mux6/1 -> Bus Creator/1  "R2X"
  Mux7/1 -> Bus Creator/2  "R2Y"
  [SM_BUS] -> Bus Selector14/1
  Bus Selector14/1 -> Mux7/2  "<R2Y>"
  [SM_BUS] -> Bus Selector17/1
  [SL_BUS] -> Bus Selector16/1
  [SL_BUS] -> Bus Selector18/1
  [SM_BUS] -> Bus Selector19/1
  [SL_BUS] -> Bus Selector20/1
  [SM_BUS] -> Bus Selector15/1
  Bus Selector16/1 -> Mux8/1  "<TH2>"
  Bus Selector17/1 -> Mux8/2  "<TH2>"
  Bus Selector18/1 -> Mux9/1  "<TH2_D>"
  Bus Selector19/1 -> Mux9/2  "<TH2_D>"
  Bus Selector20/1 -> Mux10/1  "<TH2_DD>"
  Bus Selector15/1 -> Mux10/2  "<TH2_DD>"
  Mux8/1 -> Bus Creator/8  "TH2"
  Mux9/1 -> Bus Creator/9  "TH2_DOT"
  Mux10/1 -> Bus Creator/10  "TH2_DOT_DOT"
  Ground/1 -> Bus Creator/11  "NA"

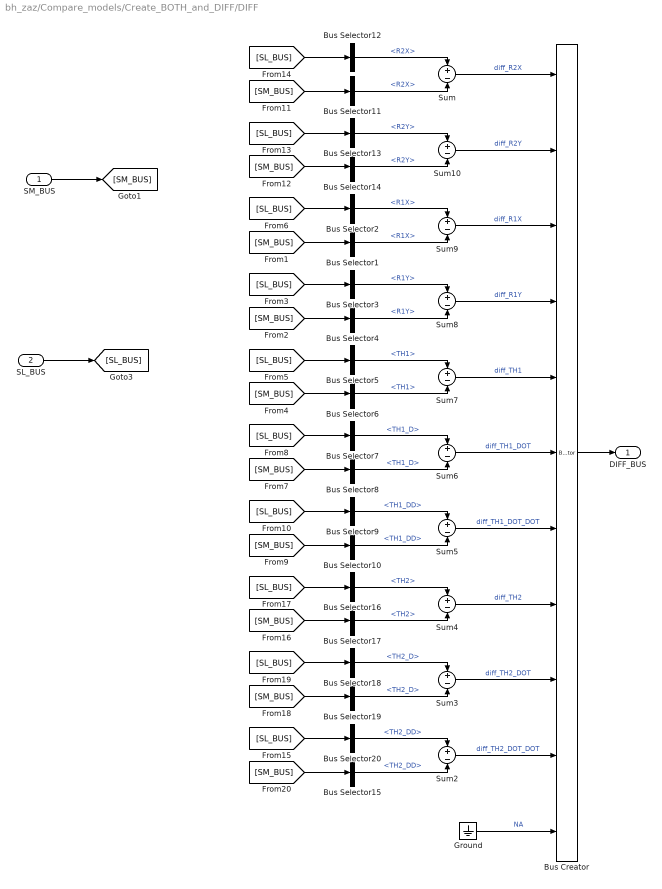
== system bh_zaz/Compare_models/Create_BOTH_and_DIFF/DIFF ==
  SM_BUS : Inport
  SL_BUS : Inport  Port=2
  Bus Creator : BusCreator  Inputs=11
  Bus Selector1 : BusSelector  OutputSignals=R1X
  Bus Selector10 : BusSelector  OutputSignals=TH1_DD
  Bus Selector11 : BusSelector  OutputSignals=R2X
  Bus Selector12 : BusSelector  OutputSignals=R2X
  Bus Selector13 : BusSelector  OutputSignals=R2Y
  Bus Selector14 : BusSelector  OutputSignals=R2Y
  Bus Selector15 : BusSelector  OutputSignals=TH2_DD
  Bus Selector16 : BusSelector  OutputSignals=TH2
  Bus Selector17 : BusSelector  OutputSignals=TH2
  Bus Selector18 : BusSelector  OutputSignals=TH2_D
  Bus Selector19 : BusSelector  OutputSignals=TH2_D
  Bus Selector2 : BusSelector  OutputSignals=R1X
  Bus Selector20 : BusSelector  OutputSignals=TH2_DD
  Bus Selector3 : BusSelector  OutputSignals=R1Y
  Bus Selector4 : BusSelector  OutputSignals=R1Y
  Bus Selector5 : BusSelector  OutputSignals=TH1
  Bus Selector6 : BusSelector  OutputSignals=TH1
  Bus Selector7 : BusSelector  OutputSignals=TH1_D
  Bus Selector8 : BusSelector  OutputSignals=TH1_D
  Bus Selector9 : BusSelector  OutputSignals=TH1_DD
  Ground : Ground
  Sum{,2..10} (10 alike) : Sum  Inputs=+|-
  DIFF_BUS : Outport
  wires:
  SL_BUS/1 -> [SL_BUS]
  SM_BUS/1 -> [SM_BUS]
  [SL_BUS] -> Bus Selector2/1
  [SM_BUS] -> Bus Selector1/1
  [SL_BUS] -> Bus Selector3/1
  [SM_BUS] -> Bus Selector4/1
  [SM_BUS] -> Bus Selector6/1
  [SL_BUS] -> Bus Selector5/1
  [SL_BUS] -> Bus Selector7/1
  [SM_BUS] -> Bus Selector8/1
  [SL_BUS] -> Bus Selector9/1
  [SM_BUS] -> Bus Selector10/1
  Bus Selector1/1 -> Sum9/2  "<R1X>"
  Bus Selector2/1 -> Sum9/1  "<R1X>"
  Bus Selector3/1 -> Sum8/1  "<R1Y>"
  Bus Selector4/1 -> Sum8/2  "<R1Y>"
  Bus Selector5/1 -> Sum7/1  "<TH1>"
  Bus Selector6/1 -> Sum7/2  "<TH1>"
  Bus Selector7/1 -> Sum6/1  "<TH1_D>"
  Bus Selector8/1 -> Sum6/2  "<TH1_D>"
  Bus Selector9/1 -> Sum5/1  "<TH1_DD>"
  Bus Selector10/1 -> Sum5/2  "<TH1_DD>"
  Sum9/1 -> Bus Creator/3  "diff_R1X"
  Sum8/1 -> Bus Creator/4  "diff_R1Y"
  Sum7/1 -> Bus Creator/5  "diff_TH1"
  Sum6/1 -> Bus Creator/6  "diff_TH1_DOT"
  Bus Creator/1 -> DIFF_BUS/1
  Sum5/1 -> Bus Creator/7  "diff_TH1_DOT_DOT"
  [SL_BUS] -> Bus Selector12/1
  [SM_BUS] -> Bus Selector11/1
  [SL_BUS] -> Bus Selector13/1
  Bus Selector11/1 -> Sum/2  "<R2X>"
  Bus Selector12/1 -> Sum/1  "<R2X>"
  Bus Selector13/1 -> Sum10/1  "<R2Y>"
  Sum/1 -> Bus Creator/1  "diff_R2X"
  Sum10/1 -> Bus Creator/2  "diff_R2Y"
  [SM_BUS] -> Bus Selector14/1
  Bus Selector14/1 -> Sum10/2  "<R2Y>"
  [SM_BUS] -> Bus Selector17/1
  [SL_BUS] -> Bus Selector16/1
  [SL_BUS] -> Bus Selector18/1
  [SM_BUS] -> Bus Selector19/1
  [SL_BUS] -> Bus Selector20/1
  [SM_BUS] -> Bus Selector15/1
  Bus Selector16/1 -> Sum4/1  "<TH2>"
  Bus Selector17/1 -> Sum4/2  "<TH2>"
  Bus Selector18/1 -> Sum3/1  "<TH2_D>"
  Bus Selector19/1 -> Sum3/2  "<TH2_D>"
  Bus Selector20/1 -> Sum2/1  "<TH2_DD>"
  Bus Selector15/1 -> Sum2/2  "<TH2_DD>"
  Sum4/1 -> Bus Creator/8  "diff_TH2"
  Sum3/1 -> Bus Creator/9  "diff_TH2_DOT"
  Sum2/1 -> Bus Creator/10  "diff_TH2_DOT_DOT"
  Ground/1 -> Bus Creator/11  "NA"

== matlab function bh_zaz/SIMULINK_MODEL/THE_THETA_SYS_DD ==
  data: I1G_s input; theta1_DD output; I2G_s input; L1X_s input; L2X_s input; g_s input; m1_s input; m2_s input; TH1D_s input; TH1_s input; TH2D_s input; TH2_s input; Q1_s input; Q2_s input; theta2_DD output
function [theta1_DD,theta2_DD] = THE_THETA_SYS_DD(I1G_s,I2G_s,L1X_s,L2X_s,g_s,m1_s,m2_s,TH1D_s,TH1_s,TH2D_s,TH2_s,Q1_s,Q2_s)
%#codegen

%    This function was generated by the Symbolic Math Toolbox version 7.1.
%    12-Dec-2016 10:22:13

theta1_DD = (I2G_s.*Q1_s.*1.6e1-I2G_s.*Q2_s.*1.6e1+L2X_s.^2.*Q1_s.*m2_s.*4.0-L2X_s.^2.*Q2_s.*m2_s.*4.0-L1X_s.*L2X_s.^2.*g_s.*m2_s.^2.*cos(TH1_s).*4.0-L1X_s.*L2X_s.*Q2_s.*m2_s.*cos(TH2_s).*8.0-I2G_s.*L1X_s.*g_s.*m1_s.*cos(TH1_s).*8.0-I2G_s.*L1X_s.*g_s.*m2_s.*cos(TH1_s).*1.6e1+L1X_s.*L2X_s.^3.*TH1D_s.^2.*m2_s.^2.*sin(TH2_s).*2.0+L1X_s.*L2X_s.^3.*TH2D_s.^2.*m2_s.^2.*sin(TH2_s).*2.0+I2G_s.*L1X_s.*L2X_s.*TH1D_s.^2.*m2_s.*sin(TH2_s).*8.0+I2G_s.*L1X_s.*L2X_s.*TH2D_s.^2.*m2_s.*sin(TH2_s).*8.0-L1X_s.*L2X_s.^2.*g_s.*m1_s.*m2_s.*cos(TH1_s).*2.0+L1X_s.*L2X_s.^3.*TH1D_s.*TH2D_s.*m2_s.^2.*sin(TH2_s).*4.0+L1X_s.*L2X_s.^2.*g_s.*m2_s.^2.*cos(TH1_s+TH2_s).*cos(TH2_s).*4.0+L1X_s.^2.*L2X_s.^2.*TH1D_s.^2.*m2_s.^2.*cos(TH2_s).*sin(TH2_s).*4.0+I2G_s.*L1X_s.*L2X_s.*TH1D_s.*TH2D_s.*m2_s.*sin(TH2_s).*1.6e1)./(I1G_s.*I2G_s.*1.6e1+L1X_s.^2.*L2X_s.^2.*m2_s.^2.*4.0+I2G_s.*L1X_s.^2.*m1_s.*4.0+I1G_s.*L2X_s.^2.*m2_s.*4.0+I2G_s.*L1X_s.^2.*m2_s.*1.6e1+L1X_s.^2.*L2X_s.^2.*m1_s.*m2_s-L1X_s.^2.*L2X_s.^2.*m2_s.^2.*cos(TH2_s).^2.*4.0);
if nargout > 1
    theta2_DD = (I1G_s.*Q2_s.*1.6e1-I2G_s.*Q1_s.*1.6e1+I2G_s.*Q2_s.*1.6e1+L1X_s.^2.*Q2_s.*m1_s.*4.0+L1X_s.^2.*Q2_s.*m2_s.*1.6e1-L2X_s.^2.*Q1_s.*m2_s.*4.0+L2X_s.^2.*Q2_s.*m2_s.*4.0-I1G_s.*L2X_s.*g_s.*m2_s.*cos(TH1_s+TH2_s).*8.0+L1X_s.*L2X_s.^2.*g_s.*m2_s.^2.*cos(TH1_s).*4.0-L1X_s.*L2X_s.*Q1_s.*m2_s.*cos(TH2_s).*8.0+L1X_s.*L2X_s.*Q2_s.*m2_s.*cos(TH2_s).*1.6e1+I2G_s.*L1X_s.*g_s.*m1_s.*cos(TH1_s).*8.0+I2G_s.*L1X_s.*g_s.*m2_s.*cos(TH1_s).*1.6e1-L1X_s.*L2X_s.^3.*TH1D_s.^2.*m2_s.^2.*sin(TH2_s).*2.0-L1X_s.^3.*L2X_s.*TH1D_s.^2.*m2_s.^2.*sin(TH2_s).*8.0-L1X_s.*L2X_s.^3.*TH2D_s.^2.*m2_s.^2.*sin(TH2_s).*2.0-L1X_s.^2.*L2X_s.*g_s.*m2_s.^2.*cos(TH1_s+TH2_s).*8.0-L1X_s.^2.*L2X_s.*g_s.*m1_s.*m2_s.*cos(TH1_s+TH2_s).*2.0-I1G_s.*L1X_s.*L2X_s.*TH1D_s.^2.*m2_s.*sin(TH2_s).*8.0-I2G_s.*L1X_s.*L2X_s.*TH1D_s.^2.*m2_s.*sin(TH2_s).*8.0-I2G_s.*L1X_s.*L2X_s.*TH2D_s.^2.*m2_s.*sin(TH2_s).*8.0+L1X_s.*L2X_s.^2.*g_s.*m1_s.*m2_s.*cos(TH1_s).*2.0-L1X_s.*L2X_s.^3.*TH1D_s.*TH2D_s.*m2_s.^2.*sin(TH2_s).*4.0-L1X_s.^3.*L2X_s.*TH1D_s.^2.*m1_s.*m2_s.*sin(TH2_s).*2.0-L1X_s.*L2X_s.^2.*g_s.*m2_s.^2.*cos(TH1_s+TH2_s).*cos(TH2_s).*4.0-L1X_s.^2.*L2X_s.^2.*TH1D_s.^2.*m2_s.^2.*cos(TH2_s).*sin(TH2_s).*8.0-L1X_s.^2.*L2X_s.^2.*TH2D_s.^2.*m2_s.^2.*cos(TH2_s).*sin(TH2_s).*4.0+L1X_s.^2.*L2X_s.*g_s.*m2_s.^2.*cos(TH1_s).*cos(TH2_s).*8.0+L1X_s.^2.*L2X_s.*g_s.*m1_s.*m2_s.*cos(TH1_s).*cos(TH2_s).*4.0-I2G_s.*L1X_s.*L2X_s.*TH1D_s.*TH2D_s.*m2_s.*sin(TH2_s).*1.6e1-L1X_s.^2.*L2X_s.^2.*TH1D_s.*TH2D_s.*m2_s.^2.*cos(TH2_s).*sin(TH2_s).*8.0)./(I1G_s.*I2G_s.*1.6e1+L1X_s.^2.*L2X_s.^2.*m2_s.^2.*4.0+I2G_s.*L1X_s.^2.*m1_s.*4.0+I1G_s.*L2X_s.^2.*m2_s.*4.0+I2G_s.*L1X_s.^2.*m2_s.*1.6e1+L1X_s.^2.*L2X_s.^2.*m1_s.*m2_s-L1X_s.^2.*L2X_s.^2.*m2_s.^2.*cos(TH2_s).^2.*4.0);
end

== matlab function bh_zaz/SIMULINK_MODEL/THE_R1_forces1 ==
  data: L1X_s input; R1_X output; m1_s input; R2X_s input; R2Y_s input; TH1DD_s input; TH1D_s input; TH1_s input; R1_Y output
function [R1_X,R1_Y] = THE_R1_forces(L1X_s,m1_s,R2X_s,R2Y_s,TH1DD_s,TH1D_s,TH1_s)
%#codegen

%    This function was generated by the Symbolic Math Toolbox version 7.0.
%    17-Aug-2016 17:09:15

R1_X = R2X_s-m1_s.*(L1X_s.*TH1D_s.^2.*cos(TH1_s).*(1.0./2.0)+L1X_s.*TH1DD_s.*sin(TH1_s).*(1.0./2.0));
if nargout > 1
    R1_Y = R2Y_s+m1_s.*(9.81e2./1.0e2)-m1_s.*(L1X_s.*TH1D_s.^2.*sin(TH1_s).*(1.0./2.0)-L1X_s.*TH1DD_s.*cos(TH1_s).*(1.0./2.0));
end

== matlab function bh_zaz/SIMULINK_MODEL/THE_R2_forces1 ==
  data: L1X_s input; R2_X output; L2X_s input; m2_s input; TH1DD_s input; TH1D_s input; TH1_s input; ALPDD_s input; ALPD_s input; ALP_s input; R2_Y output
function [R2_X,R2_Y] = THE_R2_forces(L1X_s,L2X_s,m2_s,TH1DD_s,TH1D_s,TH1_s,ALPDD_s,ALPD_s,ALP_s)
%#codegen

%    This function was generated by the Symbolic Math Toolbox version 7.0.
%    17-Aug-2016 17:09:15

R2_X = -m2_s.*(L1X_s.*TH1D_s.^2.*cos(TH1_s)+ALPDD_s.*L2X_s.*sin(ALP_s).*(1.0./2.0)+L1X_s.*TH1DD_s.*sin(TH1_s)+ALPD_s.^2.*L2X_s.*cos(ALP_s).*(1.0./2.0));
if nargout > 1
    R2_Y = m2_s.*(9.81e2./1.0e2)-m2_s.*(ALPD_s.^2.*L2X_s.*sin(ALP_s).*(1.0./2.0)+L1X_s.*TH1D_s.^2.*sin(TH1_s)-ALPDD_s.*L2X_s.*cos(ALP_s).*(1.0./2.0)-L1X_s.*TH1DD_s.*cos(TH1_s));
end
